simulink model "LKS_Controller"  (R2013b)
settings: Solver=ode45  StartTime=0.0  StopTime=3  FixedStep=1/120  MaxStep=1/120  RelTol=1e-3
model workspace (MAT data in the model file):
  Cf = 72653
  Cr = 121449
  Fy_Angle = [-20; -16; -14; -12; -10; -9.5; -9; -8.5; -8; -7.5; -7; -6.5; -6; -5.5; -5; -4.5; -4; -3.5; -3; -2.5; -2; -1.5; -1; -0.5; 0; 0.5; 1; 1.5; 2; 2.5; 3; 3.5; 4; 4.5; 5; 5.5; 6; 6.5; 7; 7.5; 8; 8.5; 9; 9.5; 10; 12; 14; 16; 18; 20]
  Fy_Data = [-1523.64 -1531.91 -1546.58 -1574.53 -1631.62 -1653.27 -1678.67 -1707.8 -1740.18 -1775.12 -1810.95 -1845.3 ... (250 elements, 50x5)]
  Fy_W = [1725 3500 6100 6950 9005]
  GearRatio = 17.25
  Izz = 3746
  Sig = Simulink.Signal
  Sig.DataType = 'auto'
  Sig.Dimensions = -1
  Sig.DimensionsMode = 'auto'
  Sig.Complexity = 'auto'
  Sig.SampleTime = -1
  Sig.SamplingMode = 'auto'
  lf = 1.17
  lr = 1.77
  m = 1820
undefined symbols (not defined in the file or in its folder): A, B, K, L
settings Model: Creator=Park  LastModifiedBy=edward
settings DataIOCC: LimitDataPoints=off  SignalLoggingSaveFormat=ModelDataLogs
settings OptimizationCC: ExpressionDepthLimit=2147483647  SimCompilerOptimization=off
settings DebuggingCC: MultiTaskDSMMsg=warning  MultiTaskCondExecSysMsg=none  FcnCallInpInsideContextMsg=UseLocalSettings  FrameProcessingCompatibilityMsg=error  StateNameClashWarn=warning
settings RTWCC: RTWCompilerOptimization=off
settings GRTTargetCC: TargetLangStandard=C89/C90 (ANSI)  CodeReplacementLibrary=None  CombineOutputUpdateFcns=off  CPPClassGenCompliant=on  GRTInterface=on
settings ConfigComp: CovMetricSettings=dw  CovHtmlReporting=on  CovSaveCumulativeToWorkspaceVar=on  CovSaveSingleToWorkspaceVar=on  CovModelRefEnable=Off  CovExternalEMLEnable=off

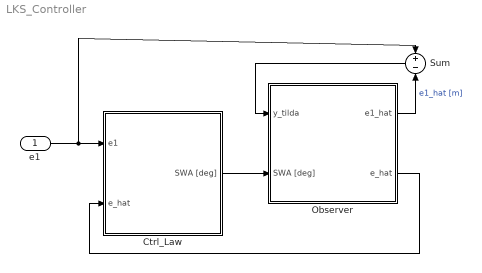
== system LKS_Controller ==
  e1 : Inport
  Ctrl_Law : Subsystem
  Observer : Subsystem
  Sum : Sum  Inputs=+-
  wires:
  Observer/2(e_hat) -> Ctrl_Law/2(e_hat)
  Ctrl_Law/1(SWA [deg]) -> Observer/2(SWA [deg])
  e1/1 -> Sum/1, Ctrl_Law/1(e1)
  Observer/1(e1_hat) -> Sum/2  "e1_hat [m]"
  Sum/1 -> Observer/1(y_tilda)

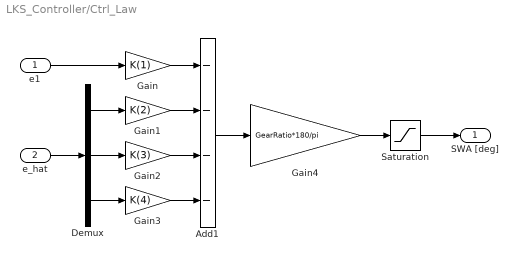
== system LKS_Controller/Ctrl_Law ==
  e1 : Inport
  e_hat : Inport  Port=2
  Add1 : Sum  Inputs=----
  Demux : Demux  Outputs=3
  Gain : Gain  Gain=K(1)
  Gain1 : Gain  Gain=K(2)
  Gain2 : Gain  Gain=K(3)
  Gain3 : Gain  Gain=K(4)
  Gain4 : Gain  Gain=GearRatio*180/pi
  Saturation : Saturate  UpperLimit=450  LowerLimit=-450
  SWA [deg] : Outport
  wires:
  Gain3/1 -> Add1/4
  Gain2/1 -> Add1/3
  Gain1/1 -> Add1/2
  Demux/3 -> Gain3/1
  Demux/2 -> Gain2/1
  Demux/1 -> Gain1/1
  e1/1 -> Gain/1
  Gain/1 -> Add1/1
  e_hat/1 -> Demux/1
  Add1/1 -> Gain4/1
  Gain4/1 -> Saturation/1
  Saturation/1 -> SWA [deg]/1

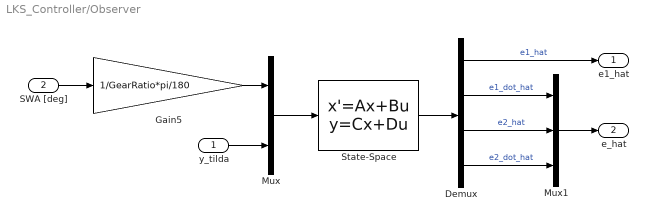
== system LKS_Controller/Observer ==
  y_tilda : Inport
  SWA [deg] : Inport  Port=2
  Demux : Demux
  Gain5 : Gain  Gain=1/GearRatio*pi/180
  Mux : Mux  Inputs=2
  Mux1 : Mux  Inputs=3
  State-Space : StateSpace  A=A  B=[B L']  C=diag([1 1 1 1])  D=zeros(4,2)  X0=0  ContinuousStateAttributes={'e1','e1_dot','e2','e2_dot'}
  e1_hat : Outport
  e_hat : Outport  Port=2
  wires:
  Mux/1 -> State-Space/1
  State-Space/1 -> Demux/1
  Demux/1 -> e1_hat/1  "e1_hat"
  y_tilda/1 -> Mux/2
  Demux/3 -> Mux1/2  "e2_hat"
  Demux/2 -> Mux1/1  "e1_dot_hat"
  Demux/4 -> Mux1/3  "e2_dot_hat"
  Mux1/1 -> e_hat/1
  SWA [deg]/1 -> Gain5/1
  Gain5/1 -> Mux/1
